simulink model "mass_damper_spring_plant"  (R2015b)
settings: Solver=VariableStepAuto  StartTime=0.0  StopTime=10.0  RelTol=1e-3
settings Model: Creator=galey  LastModifiedBy=galey

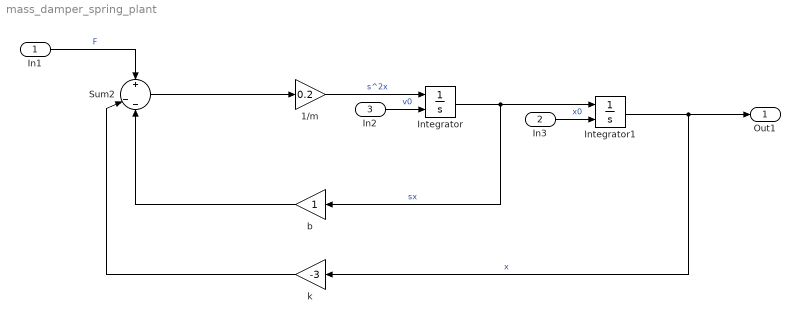
== system mass_damper_spring_plant ==
  In1 : Inport
  In3 : Inport  Port=2
  In2 : Inport  Port=3
  1/m : Gain  Gain=0.2
  Integrator : Integrator  InitialConditionSource=external
  Integrator1 : Integrator  InitialConditionSource=external
  Sum2 : Sum  Inputs=+|--
  b : Gain
  k : Gain  Gain=-3
  Out1 : Outport
  wires:
  Integrator/1 -> b/1, Integrator1/1  "sx"
  Integrator1/1 -> Out1/1, k/1  "x"
  b/1 -> Sum2/3
  In1/1 -> Sum2/1  "F"
  In2/1 -> Integrator/2  "v0"
  Sum2/1 -> 1/m/1
  1/m/1 -> Integrator/1  "s^2x"
  k/1 -> Sum2/2
  In3/1 -> Integrator1/2  "x0"
